simulink model "line_choices_snt"  (R2025b)
settings: Solver=ode45  StartTime=0.0  StopTime=10.0  RelTol=1e-3  EnableMultiTasking=on
undefined symbols (not defined in the file or in its folder): Rcouple
libraries: fl_lib x15, nesl_utility x10, ee_lib x4
settings Model: Creator=gdudgeon  LastModifiedBy=gdudgeon
settings SolverCC: AlgebraicLoopSolver=TrustRegion
settings DataIOCC: LimitDataPoints=on  SaveFormat=Array  ReturnWorkspaceOutputs=off
settings OptimizationCC: ExpressionDepthLimit=2147483647.0  LifeSpan=inf
settings DebuggingCC: UnderspecifiedInitializationDetection=Classic  MergeDetectMultiDrivingBlocksExec=none  SolverPrmCheckMsg=warning  UnconnectedInputMsg=warning  UnconnectedOutputMsg=warning  UnconnectedLineMsg=warning  StateNameClashWarn=warning  SFUnexpectedBacktrackingDiag=warning  SFNoUnconditionalDefaultTransitionDiag=warning  SFExecutionAtInitializationDiag=none  ArithmeticOperatorsInVariantConditions=warning
settings HardwareCC: ProdBitPerPointer=32.0  ProdBitPerSizeT=32.0  ProdBitPerPtrDiffT=32.0  ProdLargestAtomicFloat=None  ProdIntDivRoundTo=Undefined  ProdEndianess=Unspecified  ProdWordSize=32.0  ProdHWDeviceType=32-bit Generic
settings ModelReferenceCC: EnableRefExpFcnMdlSchedulingChecks=on  PropagateSignalLabelsOutOfModel=off
settings SFSimCC: SimUseLocalCustomCode=off  CustomCodeUndefinedFunction=UseInterfaceOnly
settings RTWCC: RTWUseLocalCustomCode=off  GPUComputeCapability=3.5
settings CodeAppCC: StateflowObjectComments=on
settings GRTTargetCC: TargetLangStandard=C89/C90 (ANSI)
settings ConfigComp: CovMetricSettings=dw  CovSaveCumulativeToWorkspaceVar=on  CovSaveSingleToWorkspaceVar=on  CovExternalEMLEnable=off  CovSFcnEnable=off
settings SimscapeCC: SimscapeNormalizeSystem=off

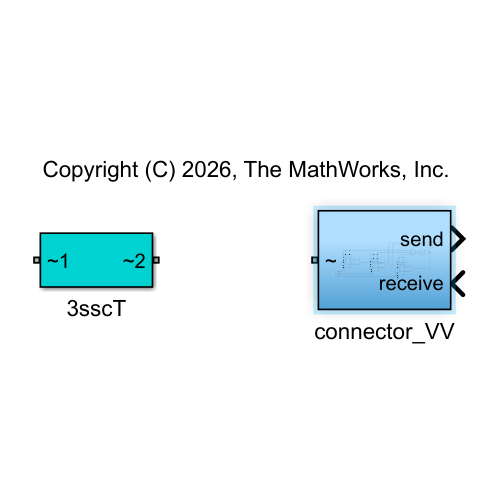
[thumbnail: Simulink's stored preview of the top-level diagram]
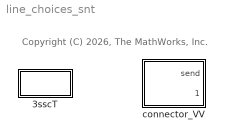
== system line_choices_snt ==
  note: Copyright (C) 2026, The MathWorks, Inc.
  3sscT : Subsystem
  connector_VV : Subsystem
      settings: PortSchema="{\"entries\":[{\"content\":{\"sides\":[{\"content\":{\"connectorIds\":[\"In1\",\"Out1\"]},\"type\":\"ConnectorPlacement.EquallySpacedRectSide\",\"uuid\":\"6f0611b6-b0cb-4818-9a76-92e90e871cd6\"},{\"content\":{\"connectorIds\":[\"RConn1\"],\"side\":\"RIGHT\"},\"type\":\"ConnectorPlacement.EquallySpacedRectSide\",\"uuid\":\"ae9441b1-f620-4671-a6ff-8cea569677fd\"},{\"content\":{\"side\":\"TOP\"},\"type\":\"ConnectorPlacement.EquallySpacedRectSide\",\"uuid\":\"4ef4c324-aa56-4a6e-b345-15c9b260ac49\"}]},\"type\":\"ConnectorPlacement.EquallySpacedConnector\",\"uuid\":\"05adf741-8513-4bc6-ade5-6cc05d9c9148\"}],\"packageUris\":[\"http://schema.mathworks.com/mf0/Connector/R2020b\"],\"version\":\"1.0\"}"

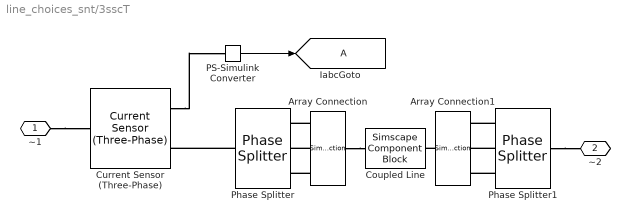
== system line_choices_snt/3sscT ==
  Array Connection : SimscapeArrayConnection  NumScalarElements=3
  Array Connection1 : SimscapeArrayConnection  NumScalarElements=3
  Coupled Line : SimscapeComponentBlock  SourceFile=multi_coupled_RL  ComponentPath=multi_coupled_RL  ComponentVariants="[\"multi_coupled_RL\"]"  ComponentVariantNames="[\"multi_coupled_RL\"]"  ClassName=multi_coupled_RL  SchemaVersion=1  noph=3  R=[1, 0, 0; 0, 1, 0; 0, 0, 1] Ohm  L=[1, 0, 0; 0, 1, 0; 0, 0, 1] H
      settings: CopyFcn=simscape.sscblock.internal.componentBlockCallback(gcbh,'COPY')  PreCopyFcn=simscape.sscblock.internal.componentBlockCallback(gcbh,'PRECOPY')  PreDeleteFcn=simscape.sscblock.internal.componentBlockCallback(gcbh,'PREDELETE')  InternalSimscapePortConfiguration="{\"Bottom\":[],\"Left\":[{\"id\":\"p\",\"label\":\"p\",\"type\":\"foundation.electrical.electrical\"}],\"Right\":[{\"id\":\"n\",\"label\":\"n\",\"type\":\"foundation.electrical.electrical\"}],\"Top\":[]}"
      mask Type: Multi-Phase Coupled RL
  Current Sensor (Three-Phase) : ee_lib/Sensors & Transducers/Current Sensor (Three-Phase)
  IabcGoto : Goto  TagVisibility=global
  PS-Simulink Converter : nesl_utility/PS-Simulink Converter  PhysicalDomain=network_engine_domain  SubClassName=ps_output  LeftPortType=input  RightPortType=output  PseudoPeriodic=off  Frequencies=[]  VectorFormat=1-D array  Unit=1  AffineConversion=off
  Phase Splitter : ee_lib/Connectors & References/Phase Splitter
  Phase Splitter1 : ee_lib/Connectors & References/Phase Splitter
  ~1 : PMIOPort  Side=Left
  ~2 : PMIOPort  Port=2  Side=Right
  wires:
  PS-Simulink Converter/1 -> IabcGoto/1
  connections:
  Phase Splitter/LConn1 -- Current Sensor (Three-Phase)/RConn2
  ~1/RConn1 -- Current Sensor (Three-Phase)/LConn1
  Current Sensor (Three-Phase)/RConn1 -- PS-Simulink Converter/LConn1
  Array Connection/RConn1 -- Coupled Line/LConn1
  Array Connection/LConn2 -- Phase Splitter/RConn2
  Array Connection/LConn1 -- Phase Splitter/RConn1
  Array Connection/LConn3 -- Phase Splitter/RConn3
  Array Connection1/RConn1 -- Coupled Line/RConn1
  Phase Splitter1/RConn3 -- Array Connection1/LConn3
  Phase Splitter1/RConn1 -- Array Connection1/LConn1
  Phase Splitter1/RConn2 -- Array Connection1/LConn2
  Phase Splitter1/LConn1 -- ~2/RConn1

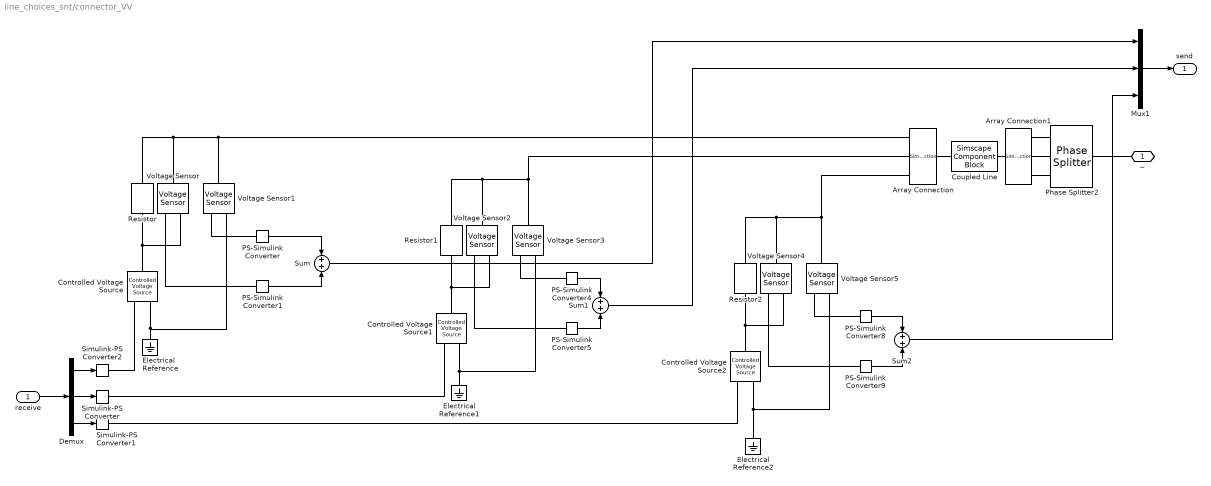
== system line_choices_snt/connector_VV ==
  receive : Inport
  Array Connection : SimscapeArrayConnection  NumScalarElements=3
  Array Connection1 : SimscapeArrayConnection  NumScalarElements=3
  Controlled Voltage Source : fl_lib/Electrical/Electrical Sources/Controlled Voltage Source
  Controlled Voltage Source1 : fl_lib/Electrical/Electrical Sources/Controlled Voltage Source
  Controlled Voltage Source2 : fl_lib/Electrical/Electrical Sources/Controlled Voltage Source
  Coupled Line : SimscapeComponentBlock  SourceFile=multi_coupled_RL  ComponentPath=multi_coupled_RL  ComponentVariants="[\"multi_coupled_RL\"]"  ComponentVariantNames="[\"multi_coupled_RL\"]"  ClassName=multi_coupled_RL  SchemaVersion=1  noph=3  R=[1, 0, 0; 0, 1, 0; 0, 0, 1] Ohm  L=[1, 0, 0; 0, 1, 0; 0, 0, 1] H
      settings: CopyFcn=simscape.sscblock.internal.componentBlockCallback(gcbh,'COPY')  PreCopyFcn=simscape.sscblock.internal.componentBlockCallback(gcbh,'PRECOPY')  PreDeleteFcn=simscape.sscblock.internal.componentBlockCallback(gcbh,'PREDELETE')  InternalSimscapePortConfiguration="{\"Bottom\":[],\"Left\":[{\"id\":\"p\",\"label\":\"p\",\"type\":\"foundation.electrical.electrical\"}],\"Right\":[{\"id\":\"n\",\"label\":\"n\",\"type\":\"foundation.electrical.electrical\"}],\"Top\":[]}"
      mask Type: Multi-Phase Coupled RL
  Demux : Demux  Outputs=3
  Electrical Reference : fl_lib/Electrical/Electrical Elements/Electrical Reference
  Electrical Reference1 : fl_lib/Electrical/Electrical Elements/Electrical Reference
  Electrical Reference2 : fl_lib/Electrical/Electrical Elements/Electrical Reference
  Mux1 : Mux  Inputs=3
  PS-Simulink Converter{,1,4..5,8..9} (6 alike) : nesl_utility/PS-Simulink Converter  PhysicalDomain=network_engine_domain  SubClassName=ps_output  LeftPortType=input  RightPortType=output  PseudoPeriodic=off  Frequencies=[]  VectorFormat=inherit  Unit=V*Hz*s  AffineConversion=off
  Phase Splitter2 : ee_lib/Connectors & References/Phase Splitter
  Resistor : fl_lib/Electrical/Electrical Elements/Resistor  R=Rcouple Ohm  i_specify=on  i_priority=Low  i=0 A  i_nominal_specify=off  i_nominal_value=1  i_nominal_unit=A  v_specify=on  v_priority=Low  v=0 V  v_nominal_specify=off  v_nominal_value=1  v_nominal_unit=V
  Resistor1 : fl_lib/Electrical/Electrical Elements/Resistor  R=Rcouple Ohm  i_specify=on  i_priority=Low  i=0 A  i_nominal_specify=off  i_nominal_value=1  i_nominal_unit=A  v_specify=on  v_priority=Low  v=0 V  v_nominal_specify=off  v_nominal_value=1  v_nominal_unit=V
  Resistor2 : fl_lib/Electrical/Electrical Elements/Resistor  R=Rcouple Ohm  i_specify=on  i_priority=Low  i=0 A  i_nominal_specify=off  i_nominal_value=1  i_nominal_unit=A  v_specify=on  v_priority=Low  v=0 V  v_nominal_specify=off  v_nominal_value=1  v_nominal_unit=V
  Simulink-PS Converter : nesl_utility/Simulink-PS Converter  PhysicalDomain=network_engine_domain  SubClassName=ps_input  LeftPortType=input  RightPortType=output  PseudoPeriodic=off  Frequencies=[]  NoiseDistribution=none  NoiseParameters=[]  Unit=1  AffineConversion=off  FilteringAndDerivatives=zero  SimscapeFilterOrder=1  InputFilterTimeConstant=0.001  UdotUserProvided=0
  Simulink-PS Converter1 : nesl_utility/Simulink-PS Converter  PhysicalDomain=network_engine_domain  SubClassName=ps_input  LeftPortType=input  RightPortType=output  PseudoPeriodic=off  Frequencies=[]  NoiseDistribution=none  NoiseParameters=[]  Unit=1  AffineConversion=off  FilteringAndDerivatives=zero  SimscapeFilterOrder=1  InputFilterTimeConstant=0.001  UdotUserProvided=0
  Simulink-PS Converter2 : nesl_utility/Simulink-PS Converter  PhysicalDomain=network_engine_domain  SubClassName=ps_input  LeftPortType=input  RightPortType=output  PseudoPeriodic=off  Frequencies=[]  NoiseDistribution=none  NoiseParameters=[]  Unit=1  AffineConversion=off  FilteringAndDerivatives=zero  SimscapeFilterOrder=1  InputFilterTimeConstant=0.001  UdotUserProvided=0
  Sum : Sum
  Sum1 : Sum
  Sum2 : Sum
  Voltage Sensor{,1..5} (6 alike) : fl_lib/Electrical/Electrical Sensors/Voltage Sensor
  ~ : PMIOPort  Side=Right
  send : Outport
  wires:
  PS-Simulink Converter5/1 -> Sum1/2
  PS-Simulink Converter1/1 -> Sum/2
  PS-Simulink Converter/1 -> Sum/1
  receive/1 -> Demux/1
  Mux1/1 -> send/1
  Demux/3 -> Simulink-PS Converter1/1
  Demux/2 -> Simulink-PS Converter/1
  Demux/1 -> Simulink-PS Converter2/1
  Sum/1 -> Mux1/1
  PS-Simulink Converter4/1 -> Sum1/1
  Sum1/1 -> Mux1/2
  PS-Simulink Converter8/1 -> Sum2/1
  PS-Simulink Converter9/1 -> Sum2/2
  Sum2/1 -> Mux1/3
  connections:
  PS-Simulink Converter8/LConn1 -- Voltage Sensor5/RConn1
  PS-Simulink Converter9/LConn1 -- Voltage Sensor4/RConn1
  Voltage Sensor5/LConn1 -- Array Connection/LConn3 -- Resistor2/LConn1 -- Voltage Sensor4/LConn1
  Controlled Voltage Source2/LConn1 -- Voltage Sensor4/RConn2 -- Resistor2/RConn1
  Controlled Voltage Source2/RConn2 -- Voltage Sensor5/RConn2 -- Electrical Reference2/LConn1
  PS-Simulink Converter5/LConn1 -- Voltage Sensor2/RConn1
  PS-Simulink Converter4/LConn1 -- Voltage Sensor3/RConn1
  Voltage Sensor2/LConn1 -- Resistor1/LConn1 -- Array Connection/LConn2 -- Voltage Sensor3/LConn1
  Controlled Voltage Source1/LConn1 -- Resistor1/RConn1 -- Voltage Sensor2/RConn2
  Controlled Voltage Source1/RConn2 -- Electrical Reference1/LConn1 -- Voltage Sensor3/RConn2
  PS-Simulink Converter/LConn1 -- Voltage Sensor1/RConn1
  PS-Simulink Converter1/LConn1 -- Voltage Sensor/RConn1
  Voltage Sensor/LConn1 -- Array Connection/LConn1 -- Voltage Sensor1/LConn1 -- Resistor/LConn1
  Controlled Voltage Source/LConn1 -- Voltage Sensor/RConn2 -- Resistor/RConn1
  Controlled Voltage Source/RConn2 -- Voltage Sensor1/RConn2 -- Electrical Reference/LConn1
  Simulink-PS Converter2/RConn1 -- Controlled Voltage Source/RConn1
  Simulink-PS Converter/RConn1 -- Controlled Voltage Source1/RConn1
  Simulink-PS Converter1/RConn1 -- Controlled Voltage Source2/RConn1
  ~/RConn1 -- Phase Splitter2/LConn1
  Phase Splitter2/RConn2 -- Array Connection1/LConn2
  Phase Splitter2/RConn1 -- Array Connection1/LConn1
  Phase Splitter2/RConn3 -- Array Connection1/LConn3
  Array Connection/RConn1 -- Coupled Line/LConn1
  Array Connection1/RConn1 -- Coupled Line/RConn1
